simulink model "grouped_signals"  (R2016a)
settings: Solver=VariableStepAuto  StartTime=0.0  StopTime=10.0  RelTol=1e-3
libraries: simulink x1
settings Model: Creator=chris.barlow  LastModifiedBy=chris.barlow

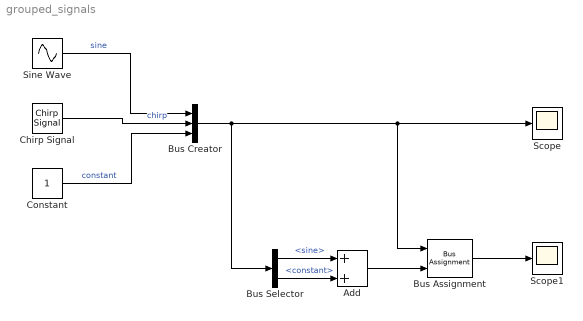
== system grouped_signals ==
  Add : Sum
  Bus Assignment : BusAssignment  AssignedSignals=sine
  Bus Creator : BusCreator  Inputs=3
  Bus Selector : BusSelector  OutputSignals=sine,constant
  Chirp Signal : simulink/Sources/Chirp Signal  f1=0.1  T=2  f2=1
  Constant : Constant
  Scope : Scope
  Scope1 : Scope
  Sine Wave : Sin  SampleTime=0
  wires:
  Sine Wave/1 -> Bus Creator/1  "sine"
  Chirp Signal/1 -> Bus Creator/2  "chirp"
  Constant/1 -> Bus Creator/3  "constant"
  Bus Creator/1 -> Bus Assignment/1, Scope/1, Bus Selector/1
  Bus Selector/1 -> Add/1  "<sine>"
  Bus Selector/2 -> Add/2  "<constant>"
  Add/1 -> Bus Assignment/2
  Bus Assignment/1 -> Scope1/1
